simulink model "helicoptertemplate"  (R2018b)
settings: Solver=ode45  StartTime=0.0  StopTime=T  RelTol=1e-3
InitFcn:
  | hwinit
values from neighbouring files (symbols this model uses):
  h = 0.02    [no_sim.m]    (also in nonlinid_helicopter.m = 0.01; test1.m = 0.01)
undefined symbols (not defined in the file or in its folder): adingain, adinoffs, HeliMexHandle
settings Model: Creator=fkzhang  LastModifiedBy=lcaric
settings DataIOCC: LimitDataPoints=on  SaveFormat=Array
settings OptimizationCC: BlockReduction=off  BooleanDataType=off  LifeSpan=inf
settings DebuggingCC: SaveWithParameterizedLinksMsg=none  UnderspecifiedInitializationDetection=Classic  MergeDetectMultiDrivingBlocksExec=none  SignalResolutionControl=TryResolveAllWithWarning  AllowSymbolicDim=off  SFUnexpectedBacktrackingDiag=warning  SFNoUnconditionalDefaultTransitionDiag=warning  SFExecutionAtInitializationDiag=none
settings HardwareCC: ProdBitPerPointer=32  ProdBitPerSizeT=32  ProdBitPerPtrDiffT=32  ProdLargestAtomicFloat=None  ProdIntDivRoundTo=Undefined  ProdEndianess=Unspecified  ProdWordSize=32  ProdHWDeviceType=32-bit Generic  TargetUnknown=on
settings ModelReferenceCC: PropagateSignalLabelsOutOfModel=off
settings SFSimCC: SimUseLocalCustomCode=off
settings RTWCC: RTWUseLocalCustomCode=off
settings CodeAppCC: StateflowObjectComments=on
settings GRTTargetCC: TargetLangStandard=C89/C90 (ANSI)  GeneratePreprocessorConditionals=Disable all
settings ConfigComp: CovMetricSettings=dw  CovHtmlReporting=on  CovSaveCumulativeToWorkspaceVar=on  CovSaveSingleToWorkspaceVar=on  CovExternalEMLEnable=off  CovSFcnEnable=off

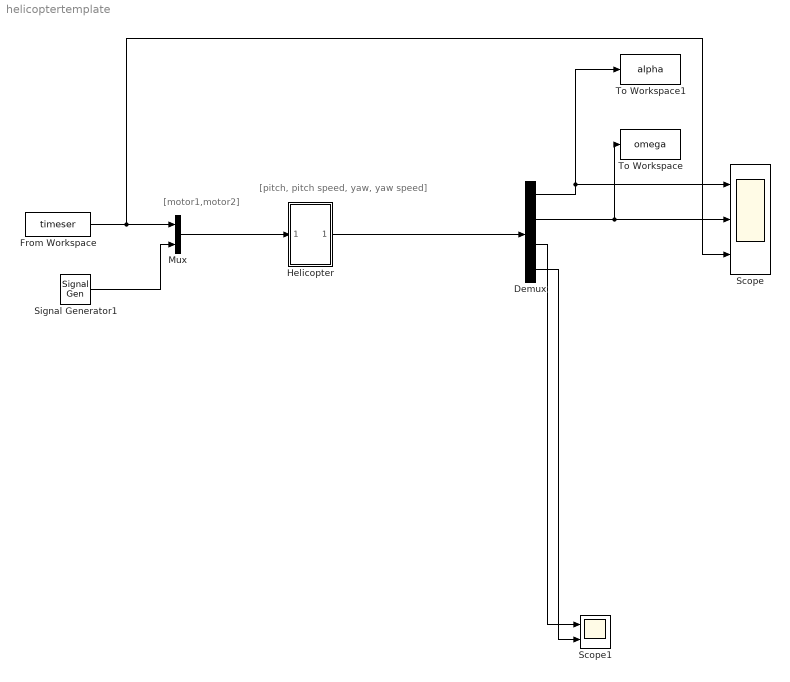
== system helicoptertemplate ==
  note: [pitch, pitch speed, yaw, yaw speed]
  note: [motor1,motor2]
  Demux : Demux
  From Workspace : FromWorkspace  VariableName=timeser  SampleTime=0
  Helicopter : Subsystem  mask{Ts=h}
      mask prompts: Ts "sampletime"
      mask init:
      | sf_heli_init
      mask Display:
      | port_label('input',1,'u');
      | port_label('output',1,'y');
  Mux : Mux  Inputs=2
  Scope : Scope  NumInputPorts=3
  Scope1 : Scope  NumInputPorts=2
  Signal Generator1 : SignalGenerator  WaveForm=square  Amplitude=0  Frequency=1/20
  To Workspace : ToWorkspace  VariableName=omega  SaveFormat=Timeseries  SampleTime=-1
  To Workspace1 : ToWorkspace  VariableName=alpha  SaveFormat=Timeseries  SampleTime=-1
  wires:
  Helicopter/1(Out1) -> Demux/1
  Demux/1 -> To Workspace1/1, Scope/1
  Mux/1 -> Helicopter/1(In1)
  Signal Generator1/1 -> Mux/2
  Demux/2 -> To Workspace/1, Scope/2
  Demux/3 -> Scope1/1
  Demux/4 -> Scope1/2
  From Workspace/1 -> Scope/3, Mux/1

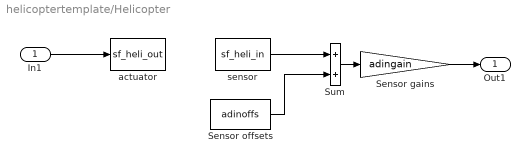
== system helicoptertemplate/Helicopter ==
  In1 : Inport
  Sensor gains : Gain  Gain=adingain
  Sensor offsets : Constant  Value=adinoffs
  Sum : Sum
  actuator : M-S-Function  FunctionName=sf_heli_out  Parameters=HeliMexHandle,Ts
  sensor : M-S-Function  FunctionName=sf_heli_in  Parameters=HeliMexHandle
  Out1 : Outport
  wires:
  sensor/1 -> Sum/1
  In1/1 -> actuator/1
  Sensor offsets/1 -> Sum/2
  Sum/1 -> Sensor gains/1
  Sensor gains/1 -> Out1/1
